simulink model "PSO_PID"  (R2024b)
settings: Solver=VariableStepAuto  StartTime=0.0  StopTime=84  FixedStep=1e-3  RelTol=1e-2
model workspace (MAT data in the model file):
  Af = 4
  Cd = 0.3
  DrCycles : object (value not decoded)
  I = 1
  Kbr = 5000
  P = 20
  TimeHWFET = 765
  TimeUDDS = 1372
  TimeUS06 = 596
  axle_b = 10
  axle_k = 5000
  bevAxle_wc = 400
  bevNp = 2
  bevNs = 30
  diffRatio = 3.4
  diffRatio1 = 3.4
  motorMaxTorqueNm = [500 500 500 500 500 500 416.666666667 357.142857143 312.5 277.777777778 250 227.272727273 ... (16 elements, 1x16)]
  motorSpeedRadPs = [0 40 80 120 160 200 240 280 320 360 400 440 ... (16 elements, 1x16)]
  vehicleMass = 1500
  wheelRadius = 0.35
undefined symbols (not defined in the file or in its folder): parms, sigbuilder_block
libraries: autolibshared x3, autolibdatasheetbattery x1, simulink x1, autolibmappedmotor x1, slpidlib x1, autolibsharedcoupling x1, autolibshareddiff x1
(part 3 of 3)

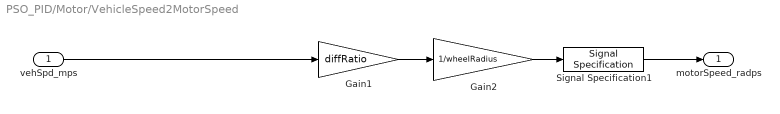
== system PSO_PID/Motor/VehicleSpeed2MotorSpeed ==
  vehSpd_mps : Inport
  Gain1 : Gain  Gain=diffRatio
  Gain2 : Gain  Gain=1/wheelRadius
  Signal Specification1 : SignalSpecification  Unit=rad/s
  motorSpeed_radps : Outport  VectorParamsAs1DForOutWhenUnconnected=off
  wires:
  Signal Specification1/1 -> motorSpeed_radps/1
  vehSpd_mps/1 -> Gain1/1
  Gain1/1 -> Gain2/1
  Gain2/1 -> Signal Specification1/1
